simulink model "cruise_control_aberta"  (R2021b)
settings: Solver=FixedStepAuto  StartTime=0.0  StopTime=100.0  FixedStep=1e-3  RelTol=1e-3
values from neighbouring files (symbols this model uses):
  b = b_car + delta_b    [closedDrag.m]    (also in identificarCruiseControl.m = f/v_inf; openDrag.m)
  d = 300    [closedDistur.m]    (also in closedDrag.m = 0; closedFf.m = 0; closedU.m = 0; closedVelRef.m = 0)
  m = tau*b    [identificarCruiseControl.m]    (also in openMass.m = m_car + m_pass)
settings Model: Creator=mmaximo  LastModifiedBy=Eric
settings SolverCC: AlgebraicLoopSolver=TrustRegion
settings DebuggingCC: SFMachineParentedDataDiag=warning

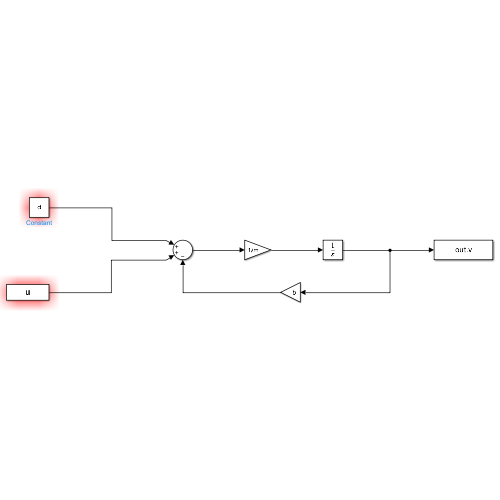
[thumbnail: Simulink's stored preview of the top-level diagram]
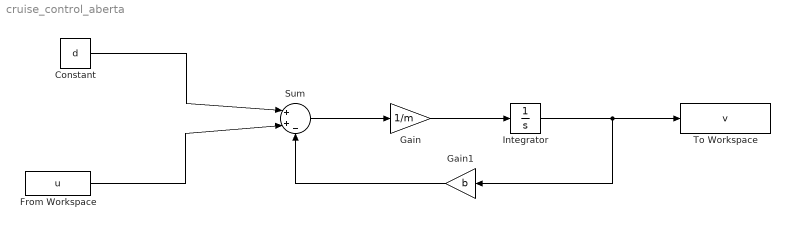
== system cruise_control_aberta ==
  Constant : Constant  Value=d
  From Workspace : FromWorkspace  VariableName=u
  Gain : Gain  Gain=1/m
  Gain1 : Gain  Gain=b
  Integrator : Integrator
  Sum : Sum  Inputs=|++-
  To Workspace : ToWorkspace  VariableName=v  SaveFormat=Structure With Time  SampleTime=-1
  wires:
  From Workspace/1 -> Sum/2
  Constant/1 -> Sum/1
  Sum/1 -> Gain/1
  Gain/1 -> Integrator/1
  Integrator/1 -> Gain1/1, To Workspace/1
  Gain1/1 -> Sum/3
